simulink model "satBFrob1"  (R2018b)
settings: Solver=VariableStepAuto  StartTime=0.0  StopTime=10.0  RelTol=1e-3
settings Model: Creator=t.lopes  LastModifiedBy=xylow
settings SFSimCC: SimUseLocalCustomCode=off
settings RTWCC: RTWUseLocalCustomCode=off

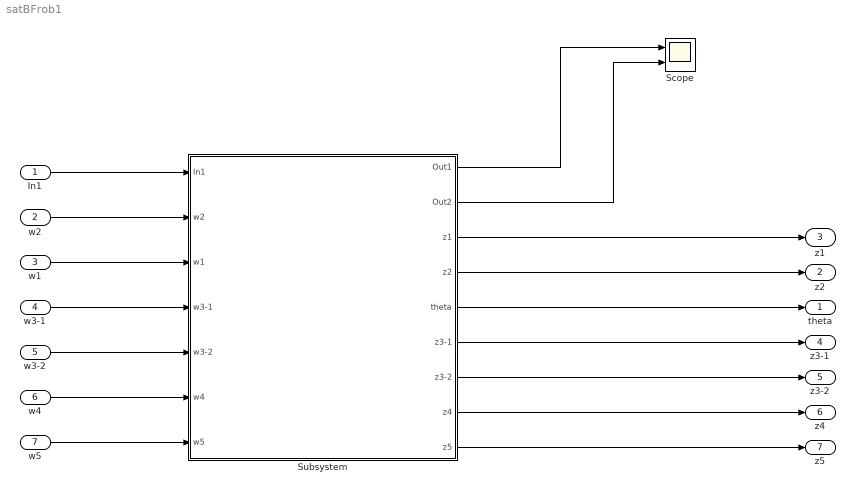
== system satBFrob1 ==
  In1 : Inport
  w2 : Inport  Port=2
  w1 : Inport  Port=3
  w3-1 : Inport  Port=4
  w3-2 : Inport  Port=5
  w4 : Inport  Port=6
  w5 : Inport  Port=7
  Scope : Scope  NumInputPorts=2
  Subsystem : Subsystem
  "theta " : Outport
  z2 : Outport  Port=2
  z1 : Outport  Port=3
  z3-1 : Outport  Port=4
  z3-2 : Outport  Port=5
  z4 : Outport  Port=6
  z5 : Outport  Port=7
  wires:
  In1/1 -> Subsystem/1(In1)
  w2/1 -> Subsystem/2(w2)
  w1/1 -> Subsystem/3(w1)
  w3-1/1 -> Subsystem/4(w3-1)
  w3-2/1 -> Subsystem/5(w3-2)
  w4/1 -> Subsystem/6(w4)
  w5/1 -> Subsystem/7(w5)
  Subsystem/1(Out1) -> Scope/1
  Subsystem/2(Out2) -> Scope/2
  Subsystem/3(z1) -> z1/1
  Subsystem/4(z2) -> z2/1
  Subsystem/5("theta ") -> "theta "/1
  Subsystem/6(z3-1) -> z3-1/1
  Subsystem/7(z3-2) -> z3-2/1
  Subsystem/8(z4) -> z4/1
  Subsystem/9(z5) -> z5/1

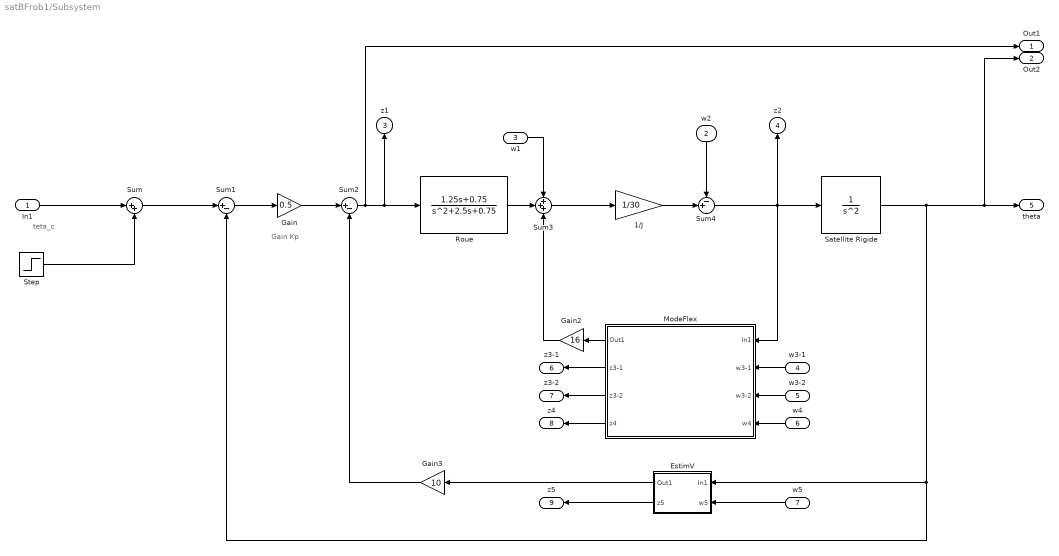
== system satBFrob1/Subsystem ==
  note: Gain Kp
  note: teta_c
  In1 : Inport
  w2 : Inport  Port=2
  w1 : Inport  Port=3
  w3-1 : Inport  Port=4
  w3-2 : Inport  Port=5
  w4 : Inport  Port=6
  w5 : Inport  Port=7
  1/J : Gain  Gain=1/30
  EstimV : Subsystem
  Gain : Gain  Gain=0.5
  Gain2 : Gain  Gain=16
  Gain3 : Gain  Gain=10
  ModeFlex : Subsystem
  Roue : TransferFcn  Numerator=[1.25 0.75]  Denominator=[1 2.5 0.75]
  Satellite Rigide : TransferFcn  Denominator=[1 0 0]
  Step : Step  After=pi/180  SampleTime=0
  Sum : Sum  Inputs=|++
  Sum1 : Sum  Inputs=|+-
  Sum2 : Sum  Inputs=|+-
  Sum3 : Sum  Inputs=+++
  Sum4 : Sum  Inputs=-+|
  Out1 : Outport
  Out2 : Outport  Port=2
  z1 : Outport  Port=3
  z2 : Outport  Port=4
  "theta " : Outport  Port=5
  z3-1 : Outport  Port=6
  z3-2 : Outport  Port=7
  z4 : Outport  Port=8
  z5 : Outport  Port=9
  wires:
  EstimV/2(z5) -> z5/1
  ModeFlex/3(z3-2) -> z3-2/1
  EstimV/1(Out1) -> Gain3/1
  w4/1 -> ModeFlex/4(w4)
  w2/1 -> Sum4/1
  ModeFlex/2(z3-1) -> z3-1/1
  Sum2/1 -> Out1/1, z1/1, Roue/1
  Sum4/1 -> z2/1, Satellite Rigide/1, ModeFlex/1(In1)
  Step/1 -> Sum/2
  ModeFlex/4(z4) -> z4/1
  w1/1 -> Sum3/1
  Sum1/1 -> Gain/1
  ModeFlex/1(Out1) -> Gain2/1
  Gain3/1 -> Sum2/2
  Satellite Rigide/1 -> "theta "/1, Out2/1, EstimV/1(In1), Sum1/2
  Sum/1 -> Sum1/1
  1/J/1 -> Sum4/2
  w3-2/1 -> ModeFlex/3(w3-2)
  Sum3/1 -> 1/J/1
  w5/1 -> EstimV/2(w5)
  Gain2/1 -> Sum3/3
  w3-1/1 -> ModeFlex/2(w3-1)
  Roue/1 -> Sum3/2
  Gain/1 -> Sum2/1
  In1/1 -> Sum/1

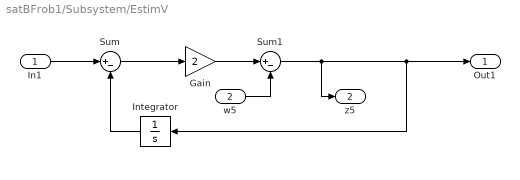
== system satBFrob1/Subsystem/EstimV ==
  In1 : Inport
  w5 : Inport  Port=2
  Gain : Gain  Gain=2
  Integrator : Integrator
  Sum : Sum  Inputs=|+-
  Sum1 : Sum  Inputs=|+-
  Out1 : Outport
  z5 : Outport  Port=2
  wires:
  Sum/1 -> Gain/1
  Integrator/1 -> Sum/2
  In1/1 -> Sum/1
  Gain/1 -> Sum1/1
  w5/1 -> Sum1/2
  Sum1/1 -> z5/1, Integrator/1, Out1/1

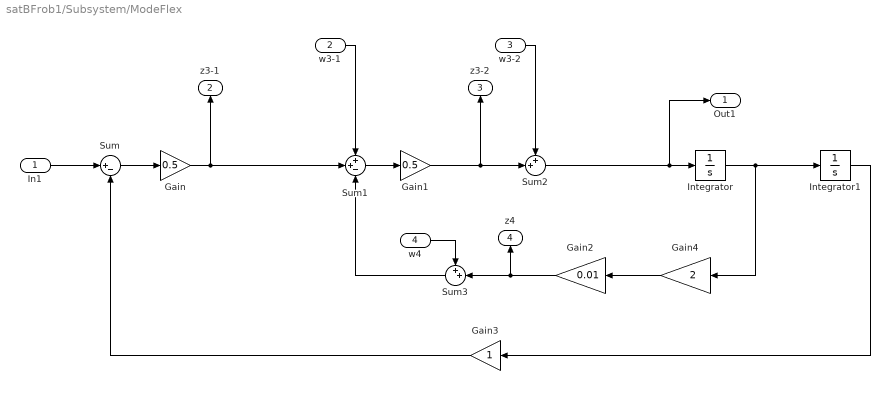
== system satBFrob1/Subsystem/ModeFlex ==
  In1 : Inport
  w3-1 : Inport  Port=2
  w3-2 : Inport  Port=3
  w4 : Inport  Port=4
  Gain : Gain  Gain=0.5
  Gain1 : Gain  Gain=0.5
  Gain2 : Gain  Gain=0.01
  Gain3 : Gain
  Gain4 : Gain  Gain=2
  Integrator : Integrator
  Integrator1 : Integrator
  Sum : Sum  Inputs=|+-
  Sum1 : Sum  Inputs=++-
  Sum2 : Sum  Inputs=++|
  Sum3 : Sum  Inputs=++|
  Out1 : Outport
  z3-1 : Outport  Port=2
  z3-2 : Outport  Port=3
  z4 : Outport  Port=4
  wires:
  In1/1 -> Sum/1
  Sum/1 -> Gain/1
  Sum1/1 -> Gain1/1
  Gain1/1 -> z3-2/1, Sum2/2
  Integrator1/1 -> Gain3/1
  Integrator/1 -> Gain4/1, Integrator1/1
  Gain3/1 -> Sum/2
  Gain4/1 -> Gain2/1
  w3-1/1 -> Sum1/1
  Gain/1 -> z3-1/1, Sum1/2
  w3-2/1 -> Sum2/1
  Sum2/1 -> Out1/1, Integrator/1
  Gain2/1 -> z4/1, Sum3/2
  Sum3/1 -> Sum1/3
  w4/1 -> Sum3/1
